simulink model "quad_standard_controllers"  (R2019b)
settings: Solver=FixedStepAuto  StartTime=0.0  StopTime=10.0  FixedStep=1/sim_freq  RelTol=1e-3
settings Model: Creator=francois  LastModifiedBy=francois
settings DebuggingCC: ModelReferenceExtraNoncontSigs=none
settings ModelReferenceCC: ModelReferenceNumInstancesAllowed=Single

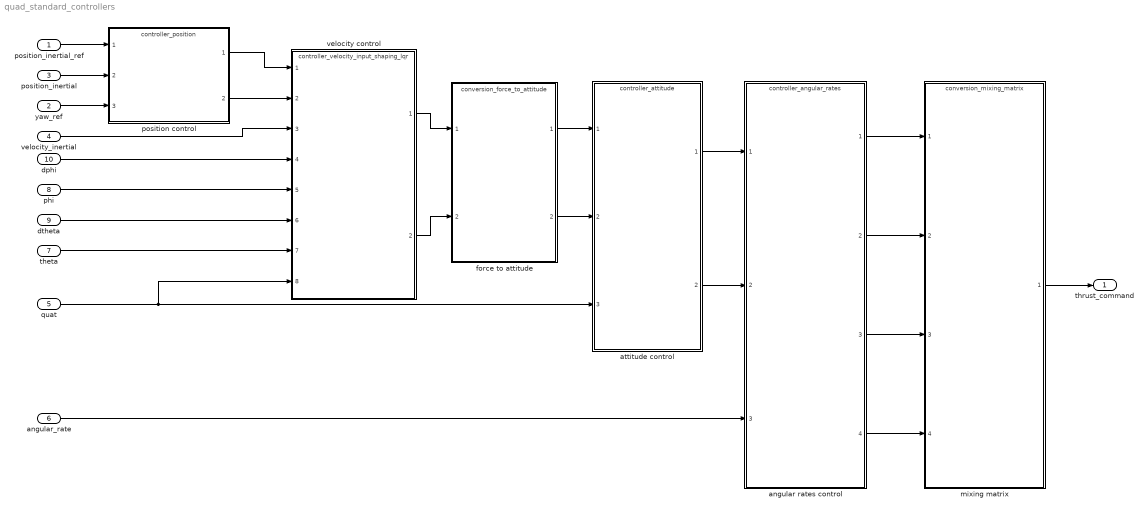
== system quad_standard_controllers ==
  position_inertial_ref : Inport
  yaw_ref : Inport  Port=2
  position_inertial : Inport  Port=3
  velocity_inertial : Inport  Port=4
  quat : Inport  Port=5  PortDimensions=4
  angular_rate : Inport  Port=6
  "theta " : Inport  Port=7
  phi : Inport  Port=8
  "dtheta " : Inport  Port=9
  dphi : Inport  Port=10
  angular rates control : ModelReference  ModelNameDialog=controller_angular_rates.slx  SimulationMode=Normal  ModelReferenceVersion=1.13
  attitude control : ModelReference  ModelNameDialog=controller_attitude.slx  SimulationMode=Normal  ModelReferenceVersion=1.16
  force to attitude : ModelReference  ModelNameDialog=conversion_force_to_attitude.slx  SimulationMode=Normal  ModelReferenceVersion=1.6
  mixing matrix : ModelReference  ModelNameDialog=conversion_mixing_matrix.slx  SimulationMode=Normal  ModelReferenceVersion=1.6
  position control : ModelReference  ModelNameDialog=controller_position.slx  SimulationMode=Normal  ModelReferenceVersion=1.5
  velocity control : ModelReference  ModelNameDialog=controller_velocity_input_shaping_lqr.slx  SimulationMode=Normal  ModelReferenceVersion=1.173
  thrust_command : Outport
  wires:
  position_inertial_ref/1 -> position control/1
  yaw_ref/1 -> position control/3
  position_inertial/1 -> position control/2
  position control/1 -> velocity control/1
  position control/2 -> velocity control/2
  velocity_inertial/1 -> velocity control/3
  velocity control/1 -> force to attitude/1
  velocity control/2 -> force to attitude/2
  force to attitude/1 -> attitude control/1
  force to attitude/2 -> attitude control/2
  quat/1 -> velocity control/8, attitude control/3
  attitude control/1 -> angular rates control/1
  attitude control/2 -> angular rates control/2
  angular_rate/1 -> angular rates control/3
  angular rates control/1 -> mixing matrix/1
  angular rates control/2 -> mixing matrix/2
  angular rates control/3 -> mixing matrix/3
  angular rates control/4 -> mixing matrix/4
  mixing matrix/1 -> thrust_command/1
  "theta "/1 -> velocity control/7
  phi/1 -> velocity control/5
  "dtheta "/1 -> velocity control/6
  dphi/1 -> velocity control/4
